simulink model "finalBS"  (R2023a)
settings: Solver=ode5  StartTime=0.0  StopTime=inf  FixedStep=0.01  RelTol=1e-3  EnableMultiTasking=on
values from neighbouring files (symbols this model uses):
  P_MAX = 38    [params.m]
  P_target_bouncy = min(P_target_bouncy, P_MAX)    [params.m]
  P_target_wood = min(P_target_wood,   P_MAX)    [params.m]
undefined symbols (not defined in the file or in its folder): DB_TICKS, FIRE_TICKS, Pmargin, TO_TICKS
libraries: arduinolib x8, slpidlib x1, simulink x1, eeGeneralControl x1, MinSegLibrary_M1V4 x1
settings Model: ExtModeTrigDuration=2  Creator=tsd7  LastModifiedBy=dangs
settings OptimizationCC: EnhancedBackFolding=on  PassReuseOutputArgsAs=Individual arguments  ZeroExternalMemoryAtStartup=off  ZeroInternalMemoryAtStartup=off  MaxStackSize=64  OptimizeBlockOrder=speed  DifferentSizesBufferReuse=on  OptimizationCustomize=off  EfficientTunableParamExpr=on
settings DebuggingCC: ParameterTunabilityLossMsg=error
settings HardwareCC: ProdBitPerInt=16  ProdBitPerPointer=16  ProdBitPerSizeT=16  ProdBitPerPtrDiffT=16  ProdLargestAtomicFloat=None  ProdWordSize=8  ProdHWDeviceType=Atmel->AVR
settings SFSimCC: MATLABDynamicMemAlloc=off
settings RTWCC: Description=Embedded Coder  SystemTargetFile=ert.tlc  HardwareBoard=Arduino Mega 2560  TemplateMakefile=ert_default_tmf  Toolchain=Arduino AVR  BuildConfiguration=Faster Runs
settings CodeAppCC: ForceParamTrailComments=on  IgnoreCustomStorageClasses=off  OperatorAnnotations=on  SimulinkDataObjDesc=on  SFDataObjDesc=on  InsertBlockDesc=on
settings ERTTargetCC: SupportContinuousTime=on  SupportVariableSizeSignals=on  ExtModeTransport=3  ExtModeStaticAlloc=on  ExtModeAutomaticAllocSize=off  ExtModeStaticAllocSize=2048  ExtModeMexFile=ext_xcp  ExtModeIntrfLevel=Level2 - Open

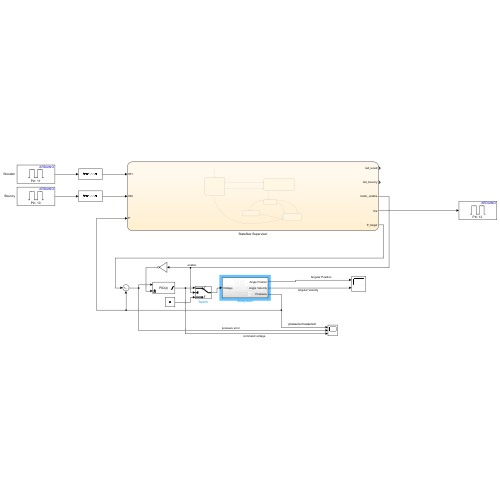
[thumbnail: Simulink's stored preview of the top-level diagram]
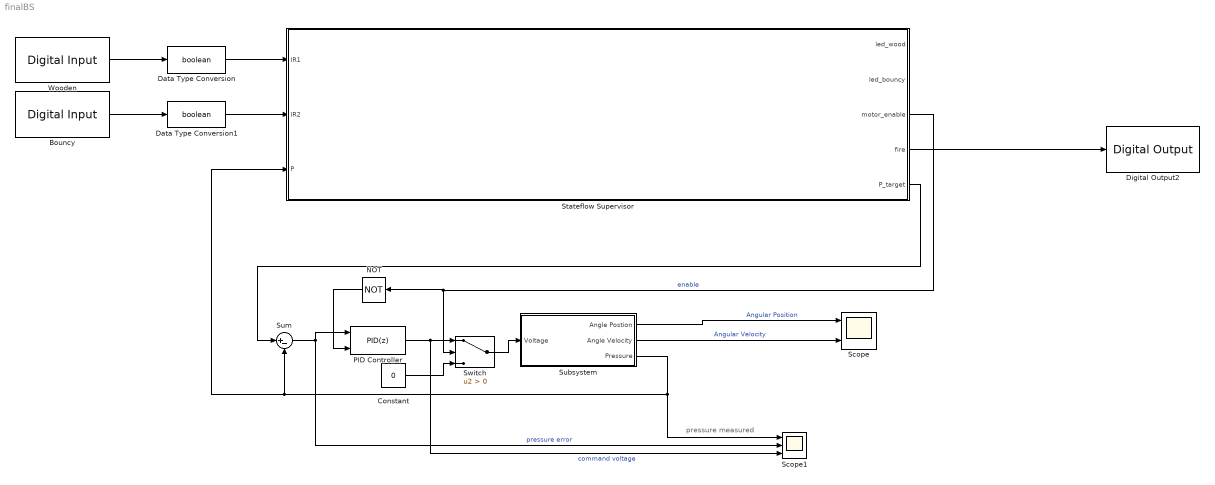
== system finalBS ==
  note: pressure measured
  Bouncy : arduinolib/Digital Input  pinNumber=10  mode=Default  Direction=input  SampleTime=0.01  blockPlatform=arduino
  Constant : Constant  Value=0
  Data Type Conversion : DataTypeConversion  OutDataTypeStr=boolean  SaturateOnIntegerOverflow=off  RndMeth=Floor
  Data Type Conversion1 : DataTypeConversion  OutDataTypeStr=boolean  SaturateOnIntegerOverflow=off  RndMeth=Floor
  Digital Output2 : arduinolib/Digital Output  pinNumber=12  Direction=output  blockPlatform=arduino
  NOT : Logic  Operator=NOT  IconShape=distinctive  AllPortsSameDT=off  OutDataTypeStr=boolean
  PID Controller : slpidlib/PID Controller  Controller=PID  Form=Parallel  TimeDomain=Discrete-time  UseExternalTs=off  SampleTime=-1  IntegratorMethod=Forward Euler  FilterMethod=Forward Euler  ControllerParametersSource=internal  P=1  I=1  UseKiTs=off  D=0  N=100  UseFilter=on  TunerSelectOption=Transfer Function Based (PID Tuner App)  InitialConditionSource=internal  InitialConditionForIntegrator=0  InitialConditionForFilter=0  DifferentiatorICPrevScaledInput=0  ExternalReset=level  TrackingMode=off  Kt=1  LimitOutput=on  SatLimitsSource=internal  UpperSaturationLimit=12  LowerSaturationLimit=-12  LinearizeAsGain=on  AntiWindupMode=clamping  Kb=1  LimitIntegrator=off  UpperIntegratorSaturationLimit=inf  LowerIntegratorSaturationLimit=-inf  POutMin=[]  POutMax=[]  IOutMin=[]  IOutMax=[]  DOutMin=[]  DOutMax=[]  NOutMin=[]  NOutMax=[]  SumOutMin=[]  SumOutMax=[]  SaturationOutMin=[]  SaturationOutMax=[]  PParamMin=[]  PParamMax=[]  IParamMin=[]  IParamMax=[]  DParamMin=[]  DParamMax=[]  NParamMin=[]  NParamMax=[]  KbParamMin=[]  KbParamMax=[]  KtParamMin=[]  KtParamMax=[]  KbOutMin=[]  KbOutMax=[]  KtOutMin=[]  KtOutMax=[]  IntegratorOutMin=[]  IntegratorOutMax=[]  FilterOutMin=[]  FilterOutMax=[]  SumI1OutMin=[]  SumI1OutMax=[]  SumI2OutMin=[]  SumI2OutMax=[]  SumI3OutMin=[]  SumI3OutMax=[]  SumI4OutMin=[]  SumI4OutMax=[]  SumDOutMin=[]  SumDOutMax=[]  DifferentiatorOutMin=[]  DifferentiatorOutMax=[]  FilterDiffOutCoefMin=[]  FilterDiffOutCoefMax=[]  ReciprocalOutMin=[]  ReciprocalOutMax=[]  SumDenOutMin=[]  SumDenOutMax=[]  SumNumOutMin=[]  SumNumOutMax=[]  DivideOutMin=[]  DivideOutMax=[]  UdiffTsProdOutMin=[]  UdiffTsProdOutMax=[]  NTsProdOutMin=[]  NTsProdOutMax=[]  UintegralTsProdOutMin=[]  UintegralTsProdOutMax=[]  UngainTsProdOutMin=[]  UngainTsProdOutMax=[]  ClampingZeroOutDataTypeStr=Inherit: Inherit via back propagation  ClampingZeroOutMin=[]  ClampingZeroOutMax=[]  FilterDenConstantOutDataTypeStr=Inherit: Inherit via back propagation  FilterDenConstantOutMin=[]  FilterDenConstantOutMax=[]  PCopyOutDataTypeStr=Inherit: Inherit via back propagation  PCopyOutMin=[]  PCopyOutMax=[]  NCopyOutDataTypeStr=Inherit: Inherit via back propagation  NCopyOutMin=[]  NCopyOutMax=[]  IntegratorContinuousStateAttributes=''  IntegratorStateMustResolveToSignalObject=off  IntegratorRTWStateStorageClass=Auto  FilterContinuousStateAttributes=''  FilterStateMustResolveToSignalObject=off  FilterRTWStateStorageClass=Auto  ParallelPVariant=InternalParameters  IdealPVariant=Disabled  IVariant=InternalParameters  DVariant=InternalParameters  IntegratorVariant=Discrete  SatVariant=Enabled  AWVariant=DiscClampingParallel  PCopyVariant=Disabled  TRVariant=Disabled  FdbkBlocksVariant=Forward  IdealPFdbkVariant=Disabled  SatFdbkVariant=Disabled  DerivativeFilterVariant=ForwardEulerFilter  NVariant=InternalParameters  NCopyVariant=Disabled  FilterICVariant=InternalICsFilter  IntegratorICVariant=InternalICs  ExternalResetVariant=ExternalReset  TRSumVariant=Passthrough  SumFdbkVariant=Disabled  SumVariant=Sum_PID  TsampFilterVariant=InternalTs  TsampNgainVariant=Passthrough  TsampIntegralVariant=Disabled_SignalSpec  ExternalSaturationOutDataTypeStr=Inherit: Same as second input
  Scope : Scope  NumInputPorts=2
  Scope1 : Scope  NumInputPorts=3
  Stateflow Supervisor : Stateflow chart  TreatAsAtomicUnit=on
  Subsystem : Subsystem
  Sum : Sum  Inputs=|+-
  Switch : Switch  Criteria=u2 > Threshold  SaturateOnIntegerOverflow=off  InputSameDT=off
  Wooden : arduinolib/Digital Input  pinNumber=11  mode=Default  Direction=input  SampleTime=0.01  blockPlatform=arduino
  wires:
  Subsystem/1(Angle Postion) -> Scope/1  "Angular Position"
  Subsystem/2(Angle Velocity) -> Scope/2  "Angular Velocity"
  Subsystem/3(Pressure) -> Scope1/1, Sum/2, Stateflow Supervisor/3(P)
  Wooden/1 -> Data Type Conversion/1
  Data Type Conversion/1 -> Stateflow Supervisor/1(IR1)
  Bouncy/1 -> Data Type Conversion1/1
  Data Type Conversion1/1 -> Stateflow Supervisor/2(IR2)
  Stateflow Supervisor/5(P_target) -> Sum/1
  Sum/1 -> Scope1/2, PID Controller/1  "pressure error"
  PID Controller/1 -> Scope1/3, Switch/1  "command voltage"
  Switch/1 -> Subsystem/1(Voltage)
  Constant/1 -> Switch/3
  Stateflow Supervisor/3(motor_enable) -> NOT/1, Switch/2  "enable"
  NOT/1 -> PID Controller/2
  Stateflow Supervisor/4(fire) -> Digital Output2/1

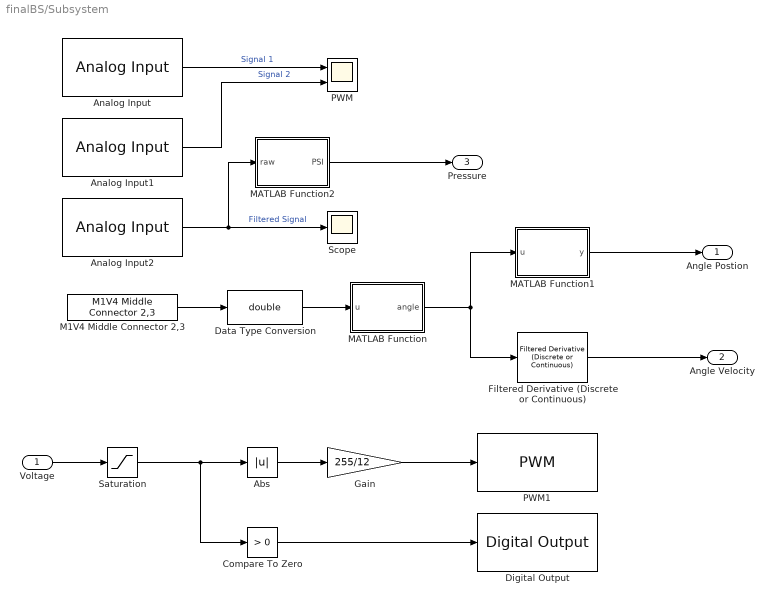
== system finalBS/Subsystem ==
  Voltage : Inport
  Abs : Abs  SaturateOnIntegerOverflow=off
  Analog Input : arduinolib/Analog Input  pinNumber=0  ReadResultsOnly=off  ConversionTriggerSource=Software  ExternalTriggerType=uint32( 0 )  OutputDataType=uint16  EnableConversionCompleteNotify=off  EnableOuputStatus=off  SampleTime=-1  blockPlatform=arduino
  Analog Input1 : arduinolib/Analog Input  pinNumber=1  ReadResultsOnly=off  ConversionTriggerSource=Software  ExternalTriggerType=uint32( 0 )  OutputDataType=uint16  EnableConversionCompleteNotify=off  EnableOuputStatus=off  SampleTime=-1  blockPlatform=arduino
  Analog Input2 : arduinolib/Analog Input  pinNumber=2  ReadResultsOnly=off  ConversionTriggerSource=Software  ExternalTriggerType=uint32( 0 )  OutputDataType=uint16  EnableConversionCompleteNotify=off  EnableOuputStatus=off  SampleTime=-1  blockPlatform=arduino
  Compare To Zero : simulink/Logic and Bit Operations/Compare To Zero  relop=>  OutDataTypeStr=boolean
  Data Type Conversion : DataTypeConversion  OutDataTypeStr=double  SaturateOnIntegerOverflow=off  RndMeth=Floor
  Digital Output : arduinolib/Digital Output  pinNumber=7  Direction=output  blockPlatform=arduino
  Filtered Derivative (Discrete or Continuous) : eeGeneralControl/Filtered Derivative (Discrete or Continuous)  K=1  T=0.1  B=inf  A=-inf  minRatio=10  init_option=Inherited from block input  x0=0  Ts=-1
      settings: LibrarySourceBlock=|
      | ee_sl_lib/General Control/Filtered Derivative
      | (Discrete or Continuous)
  Gain : Gain  Gain=255/12
  M1V4 Middle Connector 2,3 : MinSegLibrary_M1V4/M1V4 Middle Connector 2,3  Encoder=0  PinA=2  PinB=3
      settings: SourceProductName=Rensselaer Arduino Support Package
  MATLAB Function : MATLAB Function  TreatAsAtomicUnit=on
  MATLAB Function1 : MATLAB Function  TreatAsAtomicUnit=on
  MATLAB Function2 : MATLAB Function  TreatAsAtomicUnit=on
  PWM : Scope  NumInputPorts=2
  PWM1 : arduinolib/PWM  pinNumber=8  frequencyType=Default  desiredFrequency=490.2  achievableFrequency=490.2
  Saturation : Saturate  UpperLimit=12  LowerLimit=-12
  Scope : Scope
  Angle Postion : Outport
  Angle Velocity : Outport  Port=2
  Pressure : Outport  Port=3
  wires:
  Compare To Zero/1 -> Digital Output/1
  MATLAB Function/1(angle) -> MATLAB Function1/1(u), Filtered Derivative (Discrete or Continuous)/1
  Saturation/1 -> Compare To Zero/1, Abs/1
  Analog Input1/1 -> PWM/2  "Signal 2"
  Analog Input2/1 -> MATLAB Function2/1(raw), Scope/1  "Filtered Signal"
  Analog Input/1 -> PWM/1  "Signal 1"
  M1V4 Middle Connector 2,3/1 -> Data Type Conversion/1
  Gain/1 -> PWM1/1
  MATLAB Function1/1(y) -> Angle Postion/1
  Data Type Conversion/1 -> MATLAB Function/1(u)
  Abs/1 -> Gain/1
  Voltage/1 -> Saturation/1
  Filtered Derivative (Discrete or Continuous)/1 -> Angle Velocity/1
  MATLAB Function2/1(PSI) -> Pressure/1

== matlab function finalBS/Subsystem/MATLAB Function2 ==
  data: raw input; PSI output
function PSI = translation(raw)

PSI = ((raw*5/1023)/220*1000 -4)/16*100;

== matlab function finalBS/Subsystem/MATLAB Function1 ==
  data: u input; y output
function y = fcn(u)

y = mod(u, 2*pi) - pi;

== matlab function finalBS/Subsystem/MATLAB Function ==
  data: u input; angle output
function angle = count2angle(u)

N = 500; Q = 4; G = 6.3;
factor = 2 * pi / (N*Q*G);
angle = u * factor;

== stateflow chart finalBS/Stateflow Supervisor ==
  settings: updateMethod=DISCRETE  sampleTime=0.01
  state IDLE
    entry:
    led_wood = false; led_bouncy = false;
    motor_enable = false; fire = false;
    db1 = 0; db2 = 0;
    during:
    if IR1 == true
    db1 = db1 + 1;
    else
    db1 = 0;
    end
    if IR2 == true
    db2 = db2 + 1;
    else
    db2 = 0;
    end
  state DETECT
    entry:
    if type == 1
    led_wood = true;  led_bouncy = false; P_target = P_target_wood;
    else
    led_wood = false; led_bouncy = true;  P_target = P_target_bouncy;
    end
    motor_enable = true;
  state COMPRESS
    during: motor_enable = true;
  state FIRE
    entry: fire = true; motor_enable = false;
  state VENT
    entry:
    fire = false; motor_enable = false;
    led_wood = false; led_bouncy = false;
  (default) -> IDLE
  IDLE -> DETECT [order 1] : [db1 >=DB_TICKS] {type = uint8(1);}
  IDLE -> DETECT [order 2] : [db2 >= DB_TICKS]{type = uint8(2);}
  DETECT -> COMPRESS
  VENT -> IDLE : [~IR1 && ~IR2]
  COMPRESS -> FIRE [order 1] : [P >= P_target - Pmargin]
  COMPRESS -> VENT [order 2] : [P >= P_MAX]
  COMPRESS -> VENT [order 3] : after(TO_TICKS, tick)
  FIRE -> VENT : after (FIRE_TICKS, tick)
  data: IR1 input; IR2 input; P input; led_wood output; led_bouncy output; motor_enable output; fire output; P_target output; type local; db1 local; db2 local; P_target_bouncy parameter; P_target_wood parameter; Pmargin parameter; DB_TICKS parameter; FIRE_TICKS parameter; P_MAX parameter; TO_TICKS parameter
